simulink model "complete_version_no_pacer"  (Simulink 7.9)
settings: Solver=FixedStepDiscrete  StartTime=0.0  StopTime=inf  FixedStep=0.1  RelTol=1e-3
StartFcn:
  | tic
libraries: simulink x2, qbmove_library x1
settings Model: Creator=Michele  LastModifiedBy=laurentio
settings DebuggingCC: FcnCallInpInsideContextMsg=Use local settings
settings GRTTargetCC: CombineOutputUpdateFcns=off  GRTInterface=on

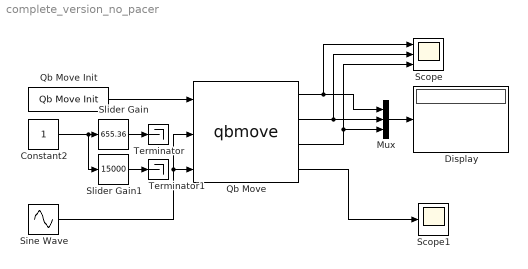
== system complete_version_no_pacer ==
  Constant2 : Constant
  Display : Display
  Mux : Mux  Inputs=3
  Qb Move : S-Function  AncestorBlock=qbmove_library/qbmove  FunctionName=qbmove  Parameters=ID, ACTIVE_COMM_DIRECTIONS, CONTROL_MODE, DAISY_CHAINING, MAX_ANG, SW_LIMIT, OFFSET  EnableBusSupport=off  mask(qb move){ID=65, ACTIVE_COMM_DIRECTIONS=Both, CONTROL_MODE=Prime Movers Positions, DAISY_CHAINING=off, MAX_ANG=0, SW_LIMIT=inf, OFFSET=0}
      mask prompts: ACTIVE_COMM_DIRECTIONS "Communication Directions"; CONTROL_MODE "Input Type"; DAISY_CHAINING "Daisy Chaining Enable"; MAX_ANG "Angle Range"; SW_LIMIT "Software Limitation of the Equilibrium Position Range"; OFFSET "Offset to the Equilibrium Position"
      mask help:
      | This block provides a interface to the Qb Move.
      | It needs an handle from Qb Move Init block.
      mask StyleString: edit,popup(Rx|Tx|Both|None),popup(Prime Movers Positions|Equilibrium Position and Stiffness Preset),checkbox,edit,edit,edit
      mask TabNameString: Options,Options,Options,Options,Options,Options,Options
      mask Display: qbmoveMaskDrawing
  Qb Move Init : qbmove_library/Qb Move Init  NUMBER_OF_COM='COM1'
  Scope : Scope  NumInputPorts=3
      settings: YMin=-1~-1~-40000  YMax=1~1~30000
  Scope1 : Scope
      settings: YMin=-1  YMax=1
  Sine Wave : Sin  Amplitude=32000  Frequency=0.5  SampleTime=0
  Slider Gain : simulink/Math Operations/Slider Gain  SystemSampleTime=-1  low=-32768  gain=655.36  high=32768
  Slider Gain1 : simulink/Math Operations/Slider Gain  SystemSampleTime=-1  low=-30000  gain=15000  high=30000
  Terminator : Terminator
  Terminator1 : Terminator
  wires:
  Constant2/1 -> Slider Gain/1, Slider Gain1/1
  Mux/1 -> Display/1
  Qb Move/1 -> Mux/1, Scope/1
  Qb Move/2 -> Scope/2, Mux/2
  Qb Move/3 -> Mux/3, Scope/3
  Qb Move/4 -> Scope1/1
  Sine Wave/1 -> Qb Move/3, Qb Move/2
  Slider Gain/1 -> Terminator/1
  Slider Gain1/1 -> Terminator1/1
  Qb Move Init/1 -> Qb Move/1
